simulink model "EV_Powertrain_Model_1_"  (R2025a)
settings: Solver=VariableStepAuto  StartTime=0.0  StopTime=20  RelTol=1e-3
libraries: simulink x1
settings Model: LastModifiedBy=maffa

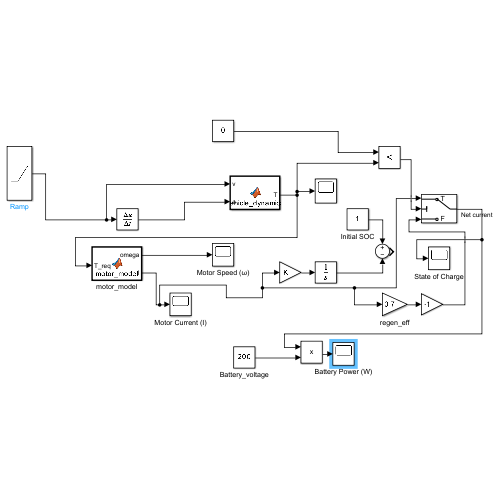
[thumbnail: Simulink's stored preview of the top-level diagram]
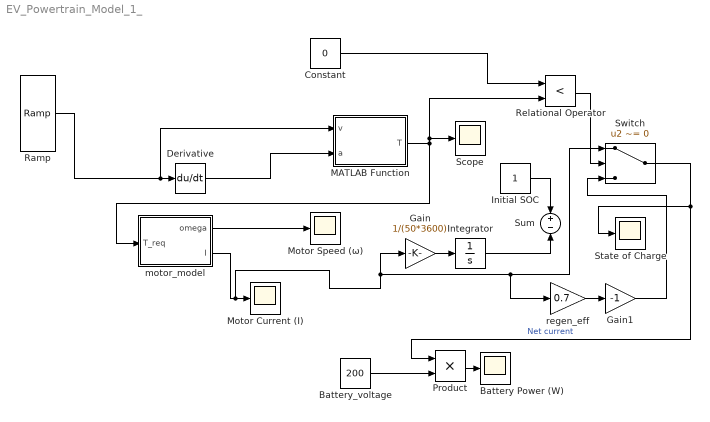
== system EV_Powertrain_Model_1_ ==
  Battery Power (W) : Scope
      settings: ActiveDisplayYMinimum=-6299.1000000000022  ActiveDisplayYMaximum=197955.90000000002  DataLoggingVariableName=ScopeData3
  Battery_voltage : Constant  Value=200
  Constant : Constant  Value=0
  Derivative : Derivative
  Gain : Gain  Gain=1/(50*3600)
  Gain1 : Gain  Gain=-1
  Initial SOC : Constant
  Integrator : Integrator
  MATLAB Function : MATLAB Function  TreatAsAtomicUnit=on
  Motor Current (I) : Scope
      settings: ActiveDisplayYMinimum=-31.495499999999993  ActiveDisplayYMaximum=989.7795000000001  DataLoggingVariableName=ScopeData2
  Motor Speed (ω) : Scope
      settings: ActiveDisplayYMinimum=402.0441  ActiveDisplayYMaximum=606.2991
  Product : Product
  Ramp : simulink/Sources/Ramp  slope=1  start=0  InitialOutput=0
  Relational Operator : RelationalOperator  Operator=<  OutDataTypeStr=boolean  RndMeth=Simplest  InputSameDT=off
  Scope : Scope
      settings: ActiveDisplayYMinimum=-1  ActiveDisplayYMaximum=1
  "State of Charge " : Scope
      settings: ActiveDisplayYMinimum=-31.495499999999993  ActiveDisplayYMaximum=989.7795000000001  DataLoggingVariableName=ScopeData4
  Sum : Sum  Inputs=+-
  Switch : Switch  Criteria=u2 ~= 0  SaturateOnIntegerOverflow=off  InputSameDT=off
  motor_model : MATLAB Function  TreatAsAtomicUnit=on
  regen_eff : Gain  Gain=0.7
  wires:
  Ramp/1 -> MATLAB Function/1(v), Derivative/1
  Derivative/1 -> MATLAB Function/2(a)
  MATLAB Function/1(T) -> Scope/1, Relational Operator/2, motor_model/1(T_req)
  motor_model/1(omega) -> Motor Speed (ω)/1
  motor_model/2(I) -> regen_eff/1, Switch/1, Gain/1, Motor Current (I)/1
  Battery_voltage/1 -> Product/2
  Product/1 -> Battery Power (W)/1
  Gain/1 -> Integrator/1
  Integrator/1 -> Sum/2
  Initial SOC/1 -> Sum/1
  Constant/1 -> Relational Operator/1
  Relational Operator/1 -> Switch/2
  regen_eff/1 -> Gain1/1
  Gain1/1 -> Switch/3
  Switch/1 -> Product/1, "State of Charge "/1  "Net current"

== matlab function EV_Powertrain_Model_1_/MATLAB Function ==
  data: v input; a input; T output
function T = vehicle_dynamics(v, a)
    m = 1200; g = 9.81; Cr = 0.01;
    rho = 1.225; A = 2.2; Cd = 0.3; R = 0.3;
    F_inertia = m * a;
    F_roll    = m * g * Cr;
    F_aero    = 0.5 * rho * A * Cd * v^2;
    T = (F_inertia + F_roll + F_aero) * R;
end

== matlab function EV_Powertrain_Model_1_/motor_model ==
  data: T_req input; omega output; I output
function [omega, I] = motor_model(T_req)
    % Motor parameters
    Kt = 0.5;    % Nm/A
    Ke = 0.5;    % V·s/rad
    Rm = 0.1;    % Ohm (winding resistance)
    J  = 0.1;    % kg·m^2 (rotor inertia)
    Vb = 300;    % V (battery voltage)

    % Current needed to produce torque
    I = T_req / Kt;

    % Electrical voltage after resistive drop
    V_emf = Vb - I * Rm;

    % Angular speed from back-EMF constant
    omega = V_emf / Ke;
end
